simulink model "skuska"  (R2023b)
settings: Solver=VariableStepAuto  StartTime=0.0  StopTime=20  RelTol=1e-3
values from neighbouring files (symbols this model uses):
  A = double(A_linear)    [main.m]    (also in rlqr.m = [0 1; -6 -5])
  B = double(B_linear)    [main.m]    (also in rlqr.m = [0;1])
  C = eye(2)    [main.m]    (also in rlqr.m)
undefined symbols (not defined in the file or in its folder): K1
settings Model: Creator=ralex  LastModifiedBy=ralex

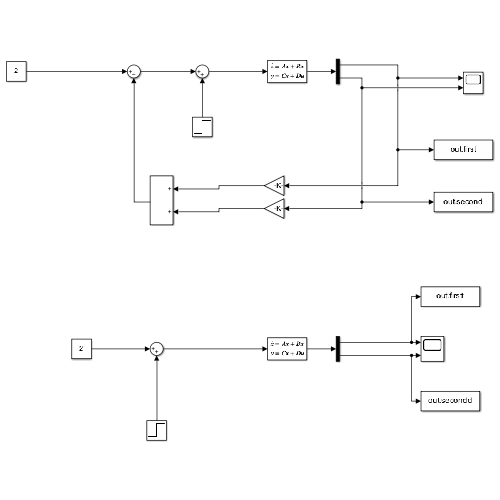
[thumbnail: Simulink's stored preview of the top-level diagram]
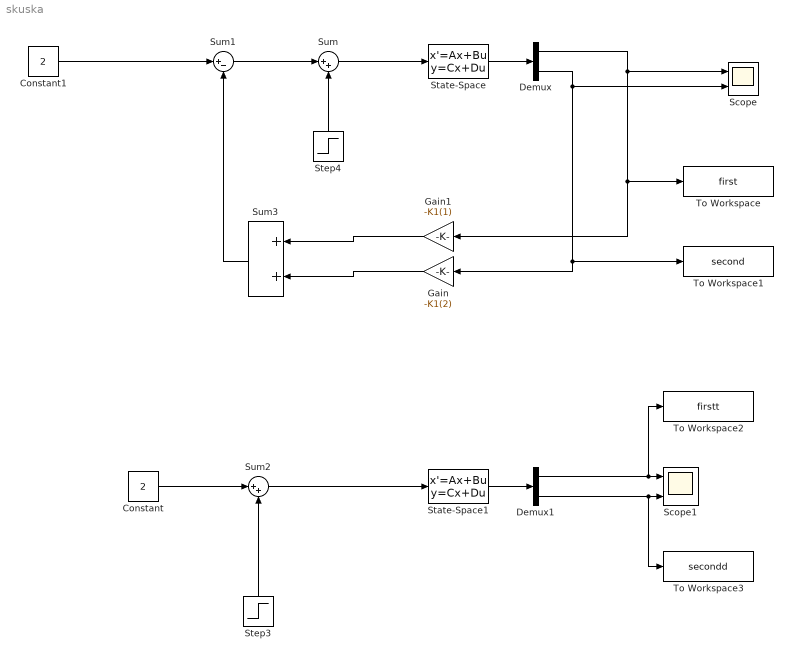
== system skuska ==
  Constant : Constant  Value=2
  Constant1 : Constant  Value=2
  Demux : Demux  Outputs=2
  Demux1 : Demux  Outputs=2
  Gain : Gain  Gain=-K1(2)
  Gain1 : Gain  Gain=-K1(1)
  Scope : Scope  NumInputPorts=2
  Scope1 : Scope  NumInputPorts=2
  State-Space : StateSpace  A=A  B=B  C=eye(2)  D=[0;0]  InitialCondition=[0 0]
  State-Space1 : StateSpace  A=A  B=B  C=C  D=[0;0]  InitialCondition=[0 0]
  Step3 : Step  Time=10  Before=2  After=3  SampleTime=0
  Step4 : Step  Time=10  Before=2  After=3  SampleTime=0
  Sum : Sum  Inputs=|++
  Sum1 : Sum  Inputs=|+-
  Sum2 : Sum  Inputs=|++
  Sum3 : Sum
  To Workspace : ToWorkspace  VariableName=first  SaveFormat=Timeseries  SampleTime=-1
  To Workspace1 : ToWorkspace  VariableName=second  SaveFormat=Timeseries  SampleTime=-1
  To Workspace2 : ToWorkspace  VariableName=firstt  SaveFormat=Timeseries  SampleTime=-1
  To Workspace3 : ToWorkspace  VariableName=secondd  SaveFormat=Timeseries  SampleTime=-1
  wires:
  Demux/2 -> Gain/1, To Workspace1/1, Scope/2
  State-Space/1 -> Demux/1
  Demux/1 -> Gain1/1, To Workspace/1, Scope/1
  State-Space1/1 -> Demux1/1
  Demux1/1 -> To Workspace2/1, Scope1/1
  Demux1/2 -> To Workspace3/1, Scope1/2
  Sum1/1 -> Sum/1
  Sum/1 -> State-Space/1
  Sum2/1 -> State-Space1/1
  Constant/1 -> Sum2/1
  Constant1/1 -> Sum1/1
  Gain1/1 -> Sum3/1
  Gain/1 -> Sum3/2
  Sum3/1 -> Sum1/2
  Step4/1 -> Sum/2
  Step3/1 -> Sum2/2
